simulink library "lib_TCML"  (R2015a)
settings: Solver=ode45  StartTime=0.0  StopTime=10.0  RelTol=1e-3
libraries: simulink x5
(part 6 of 7)

== matlab function lib_TCML/Dynamic Tip Clearance/Case Deformation/1D Trans Conduction model - variable props & general BCs/MATLAB Function ==
  data: k input; T output; Cp input; rho input; convin input; Tfin input; hin input; condin input; Tsin input; radin input; Textin input; uin input; convout input; Tfout input; hout input; condout input; Tsout input; radout input; Textout input; uout input; x input; a input; dt input; To input; Erro input; Err output; BN input
function [T,Err] = HeatX1D(k,Cp,rho,convin,Tfin,hin,condin,Tsin,...
    radin,Textin,uin,convout,Tfout,hout,condout,Tsout,radout,Textout,uout,...
    x,a,dt,To,Erro,BN)
%#codegen

% Written by: Jonathan Kratz, NASA GRC
% Date: August 1, 2016
%
% Description: This MATLAB function block solves a 1-D heat transfer
% problem with the potential for various boundary conditions including
% convection, conduction, and radiation. The function is capable of
% accepting time-varying thermal properties including the conductivity,
% specific heat, and density of the solid structure. Heat transfer
% coefficients can also be time-varying. The function is equiped to handle
% planor and cylindrical geometries. A generic non-uniform spatial
% discretization may be used but a constant time-step is encouraged for
% accuracy in time. The block applies a 1-D Finite Difference Method (FDM)
% to solve the equation:
%                  _                     _
%   dT     1      |  /dk   ak\ dT     d2T |
%   -- = ------ * | | -- + -- |-- + k --- |
%   dt   rho*Cp   |_ \dx    x/ dx     dx2_|
%
% This is done through the Crank-Nicolson Method in conjunction with 
% Thomas's Algorithm. The boundary conditions use linear heat transfer 
% coefficients and it is suggested that these coefficients be evaluated 
% using thermal properties of the previous time-step (i.e. temperature of 
% the structure and thermodynamic properties of the surrounding gases).
% Depending on the problem they may be assumed constant.
%
% Inputs:
% Thermal Properties:
%   k - thermal conductivity of the structure [1 x number of nodes]
%   Cp - heat capacity of the structure [1 x number of nodes]
%   rho - density of the structure [1 x number of nodes]
% Boundary Conditions:
%   Tfin - temperature of fluid on the inside surface
%   hin - convective heat transfer coefficient on the inside surface
%   Tsin - temperature of a contacting structure on the inside surface
%   Textin - temperature of a distant external radiating source/sink 
%       exposed to the inner surface
%   uin - linear radiative heat transfer coefficient between the inner
%       surface and external radiating source/sink it is exposed to
%   Tfout - temperature of fluid on the outer surface
%   hout - convective heat transfer coefficient on the outer surface
%   Tsout - temperature of a contacting structure on the outer surface
%   Textout - temperature of a distant external radiating source/sink 
%       exposed to the outer surface
%   uin - linear radiative heat transfer coefficient between the outer
%       surface and external radiating source/sink it is exposed to
% Geometry/Discretization:
%   x - discretized spatial coordinates
%   a - shape variable (0 - planar, 1 - cylindrical)
% Solver:
%   dt - time-step of the solver
%   To - initial condition for the solver/initial temperature of the
%       structure [1 x number of nodes]
% Error/Warning Detection
%   Erro - array with error states. Tracks errors/warnings that have been
%       detected.
%   BN - block name. Used in warning messages.
%  
% Discretization guidelines: The first and last nodes should be on the 
% surface. It is important that that the first node should be half the size 
% as the second node and the last node should be half the size of the 
% second to last node. This is due to the assumptions made in the 
% formulization of the boundary condition equations. Also, for planar 
% geometries the first value of the discretization array x (which 
% corresponds to the first node) can be any real numeric value (it does not
% have to be zero, equations use node size so relative position is what 
% matters). In the case of a cylindrical geometry the first value in the x 
% array should be the inner radius of the structure. It should go without 
% saying that the spatial discretization array x is required to be 
% montonically increasing.

% number of elements
n = length(x); %number of nodes

% initialize error/warning array
Err = Erro;
ErrNum = 1; %Error index

% check sizes ------------------------------------------------------------%
if length(x) < 4 && Erro(ErrNum) == 0
    Err(ErrNum) = 1;
    fprintf('warning in %s: x must be an array of length > 3\n',char(BN));
end
ErrNum = ErrNum + 1;
if length(k) ~= length(x) && Erro(ErrNum) == 0
    Err(ErrNum) = 1;
    fprintf('warning in %s: length of k must equal length of x\n',char(BN));
end
ErrNum = ErrNum + 1;
if length(Cp) ~= length(x) && Erro(ErrNum) == 0
    Err(ErrNum) = 1;
    fprintf('warning in %s: length of k must equal length of x\n',char(BN));
end
ErrNum = ErrNum + 1;
if length(rho) ~= length(x) && Erro(ErrNum) == 0
    Err(ErrNum) = 1;
    fprintf('warning in %s: length of k must equal length of x\n',char(BN));
end
ErrNum = ErrNum + 1;
if length(x) ~= length(x) && Erro(ErrNum) == 0
    Err(ErrNum) = 1;
    fprintf('warning in %s: length of k must equal length of x\n',char(BN));
end
ErrNum = ErrNum + 1;
if length(Tfin) ~= 1 && Erro(ErrNum) == 0
    Err(ErrNum) = 1;
    fprintf('warning in %s: Tfin must be a scalar\n',char(BN));
end
ErrNum = ErrNum + 1;
if length(hin) ~= 1 && Erro(ErrNum) == 0
    Err(ErrNum) = 1;
    fprintf('warning in %s: hin must be a scalar\n',char(BN));
end
ErrNum = ErrNum + 1;
if length(Tsin) ~= 1 && Erro(ErrNum) == 0
    Err(ErrNum) = 1;
    fprintf('warning in %s: Tsin must be a scalar\n',char(BN));
end
ErrNum = ErrNum + 1;
if length(Textin) ~= 1 && Erro(ErrNum) == 0
    Err(ErrNum) = 1;
    fprintf('warning in %s: Textin must be a scalar\n',char(BN));
end
ErrNum = ErrNum + 1;
if length(uin) ~= 1 && Erro(ErrNum) == 0
    Err(ErrNum) = 1;
    fprintf('warning in %s: uin must be a scalar\n',char(BN));
end
ErrNum = ErrNum + 1;
if length(Tfout) ~= 1 && Erro(ErrNum) == 0
    Err(ErrNum) = 1;
    fprintf('warning in %s: Tfout must be a scalar\n',char(BN));
end
ErrNum = ErrNum + 1;
if length(hout) ~= 1 && Erro(ErrNum) == 0
    Err(ErrNum) = 1;
    fprintf('warning in %s: hout must be a scalar\n',char(BN));
end
ErrNum = ErrNum + 1;
if length(Tsout) ~= 1 && Erro(ErrNum) == 0
    Err(ErrNum) = 1;
    fprintf('warning in %s: Tsout must be a scalar\n',char(BN));
end
ErrNum = ErrNum + 1;
if length(Textout) ~= 1 && Erro(ErrNum) == 0
    Err(ErrNum) = 1;
    fprintf('warning in %s: Textout must be a scalar\n',char(BN));
end
ErrNum = ErrNum + 1;
if length(uout) ~= 1 && Erro(ErrNum) == 0
    Err(ErrNum) = 1;
    fprintf('warning in %s: uin must be a scalar\n',char(BN));
end
ErrNum = ErrNum + 1;
if ((length(a) ~= 1) || (a ~= 0 && a ~= 1)) && Erro(ErrNum) == 0
    Err(ErrNum) = 1;
    fprintf('warning in %s: a must be a scalar equal to 0 or 1\n',char(BN));
end
ErrNum = ErrNum + 1;
if (length(dt) ~= 1 || dt <= 0) && Erro(ErrNum) == 0
    Err(ErrNum) = 1;
    fprintf('warning in %s: dt must be a positive scalar\n',char(BN));
end
ErrNum = ErrNum + 1;

% check for physical impossibilities
if min(k) <= 0 && Erro(ErrNum) == 0
    Err(ErrNum) = 1;
    fprintf('warning in %s: elements of k cannot be zero or negative\n',char(BN));
end
ErrNum = ErrNum + 1;
if min(Cp) <= 0 && Erro(ErrNum) == 0
    Err(ErrNum) = 1;
    fprintf('warning in %s: elements of Cp cannot be zero or negative\n',char(BN));
end
ErrNum = ErrNum + 1;
if min(rho) <= 0 && Erro(ErrNum) == 0
    Err(ErrNum) = 1;
    fprintf('warning in %s: elements of rho cannot be zero or negative\n',char(BN));
end
ErrNum = ErrNum + 1;
if min(To) < 0 && Erro(ErrNum) == 0
    Err(ErrNum) = 1;
    fprintf('warning in %s: elements of T0 are negative. On an absolute scale this is not possible.\n',char(BN));
end
ErrNum = ErrNum + 1;
if Tfin < 0 && Erro(ErrNum) == 0
    Err(ErrNum) = 1;
    fprintf('warning in %s: Tfin is negative. On an absolute scale this is not possible.\n',char(BN));
end
ErrNum = ErrNum + 1;
if Tfout < 0 && Erro(ErrNum) == 0
    Err(ErrNum) = 1;
    fprintf('warning in %s: Tfout is negative. On an absolute scale this is not possible.\n',char(BN));
end
ErrNum = ErrNum + 1;
if Tsin < 0 && Erro(ErrNum) == 0
    Err(ErrNum) = 1;
    fprintf('warning in %s: Tsin is negative. On an absolute scale this is not possible.\n',char(BN));
end
ErrNum = ErrNum + 1;
if Tsout < 0 && Erro(ErrNum) == 0
    Err(ErrNum) = 1;
    fprintf('warning in %s: Tsout is negative. On an absolute scale this is not possible.\n',char(BN));
end
ErrNum = ErrNum + 1;
if Textin < 0 && Erro(ErrNum) == 0
    Err(ErrNum) = 1;
    fprintf('warning in %s: Textin is negative. On an absolute scale this is not possible.\n',char(BN));
end
ErrNum = ErrNum + 1;
if Textout < 0 && Erro(ErrNum) == 0
    Err(ErrNum) = 1;
    fprintf('warning in %s: Textout is negative. On an absolute scale this is not possible.\n',char(BN));
end
ErrNum = ErrNum + 1;
if hin < 0 && Erro(ErrNum) == 0
    Err(ErrNum) = 1;
    fprintf('warning in %s: hin must be positive.\n',char(BN));
end
ErrNum = ErrNum + 1;
if hout < 0 && Erro(ErrNum) == 0
    Err(ErrNum) = 1;
    fprintf('warning in %s: hout must be positive.\n',char(BN));
end
ErrNum = ErrNum + 1;
if uin < 0 && Erro(ErrNum) == 0
    Err(ErrNum) = 1;
    fprintf('warning in %s: uin must be positive.\n',char(BN));
end
ErrNum = ErrNum + 1;
if uout < 0 && Erro(ErrNum) == 0
    Err(ErrNum) = 1;
    fprintf('warning in %s: uout must be positive.\n',char(BN));
end
ErrNum = ErrNum + 1;

% check for defiance of block constraints
diffx = diff(x);
if min(diffx) <= 0 && Erro(ErrNum) == 0
    Err(ErrNum) = 1;
    fprintf('warning in %s: x must be monotonically increasing\n',char(BN));
end
ErrNum = ErrNum + 1;
if (x(2)-x(1))-(x(3)-x(2)) >= 10^-5 && Erro(ErrNum) == 0
    Err(ErrNum) = 1;
    fprintf('warning in %s: the first node may not be half the thickness of the\nneighboring interior node as is required for planar geometries in the\nequation formulation of this block. To assure the first node is\nof the appropriate size assure (x(2)-x(1))-(x(3)-x(2)) = 0.\n',char(BN));
end
ErrNum = ErrNum + 1;
if (x(n)-x(n-1))-(x(n-1)-x(n-2)) >= 10^-5 && Erro(ErrNum) == 0
    Err(ErrNum) = 1;
    fprintf('warning in %s: the last node may not be half the thickness of the\nneighboring interior node as is required for planar geometries in the\nequation formulation of this block. To assure the last node is\nof the appropriate size assure (x(n)-x(n-1))-(x(n-1)-x(n-2)) = 0\nwhere n is the total number of nodes.\n',char(BN));
end
ErrNum = ErrNum + 1;
if a == 1 && x(1) < 10^-6 %protect against dividing by zero
    if Erro(ErrNum) == 0
        fprintf('warning in %s: x(1) is close to zero, value changed to 10^-6 to prevent dividing by zero\n',char(BN));
    end
    Err(ErrNum) = 1;
    x(1) = 10^-6;
end
ErrNum = ErrNum + 1;

% verify at least one BC type is active for each surface
if condin == 0 && convin == 0 && radin == 0 && Erro(ErrNum) == 0
    fprintf('warning in %s: at least one boundary condition type (convection, radiation, conduction) must be active for the inner surface\n',char(BN));
    Err(ErrNum) = 1;
end
ErrNum = ErrNum + 1;
% verify at least one BC type is active for each surface
if condout == 0 && convout == 0 && radout == 0 && Erro(ErrNum) == 0
    fprintf('warning in %s: at least one boundary condition type (convection, radiation, conduction) must be active for the outer surface\n',char(BN));
    Err(ErrNum) = 1;
end

% make external convection at boundaries zero if there is no convection BC
if convin == 0
    hin = 0;
end
if convout == 0
    hout = 0;
end

% make external radiation at boundaries zero if there is no radiation BC
if radin == 0
    uin = 0;
end
if radout == 0
    uout = 0;
end

% form system of equations in tridiagonal arrays -------------------------%
%  _                                 _  _   _     _   _ 
% | D1   A1   0    .    .    .    0   || T1  |   | C1  |
% | B1   D2   A2   0              .   || T2  |   | C2  |
% | 0    B2   D3   A3   .         .   || T3  |   | C3  |
% | .    0    .    .    .    .    .   || .   | = | .   |
% | .         .    .    .    .    0   || .   |   | .   | 
% | .              .    Bn-2 Dn-1 An-1|| Tn-1|   | Cn-1|
% |_0    .    .    .    0    Bn-1 Dn _||_Tn _|   |_Cn _|
%
% Initialize system arrays B, D, A, and C
B = zeros(1,n); %initialize B array
D = zeros(1,n); %initialize D array
A = zeros(1,n); %initialize A array
C = zeros(1,n); %initialize C array
% node thickness
dx = zeros(1,n); %initialize dx array
for i = 1:n
    if i == 1
        dx(i) = (x(2)-x(1));
    elseif i == n
        dx(i) = (x(n)-x(n-1));
    else
        del1 = x(i) - x(i-1);
        dx(i) = 2*del1 - dx(i-1);
    end
end
% --- inner node (half size of interior node with point on surface)
Fo1 = 0; %Fourier number
Bi1 = 0; %Boit number
BiRad1 = 0; %analogous Boit number for radiation
Fos1 = 0; %Fourier number for conduction BC
dx1 = x(2) - x(1); %node size
% planar
if a == 0
    Fo1 = dt*k(1)/(rho(1)*Cp(1)*dx1^2); %Fourier number
    Bi1 = hin*dx1/k(1); %Boit number
    BiRad1 = uin*dx1/k(1); %analogous Boit number for radiation
    if condin == 0
        Fos1 = 0;
    else
        Fos1 = Fo1; %Fourier number for conduction BC
    end
end
% cylindrical
if a == 1
    Fo1 = dt*k(1)/(rho(1)*Cp(1)*((x(2)-dx1/2)^2-x(1)^2)*log(x(2)/x(1))); %Fourier number
    Bi1 = hin*x(1)*log(x(2)/x(1))/k(1); %Boit number
    BiRad1 = uin*x(1)*log(x(2)/x(1))/k(1); %analogous Boit number for radiation
    if condin == 0
        Fos1 = 0;
    else
        if (x(1)-dx1) <= 0
            dx1 = 0;
        end
        Fos1 = dt*k(1)/(rho(1)*Cp(1)*((x(2)-dx1/2)^2-x(1)^2)*log((x(1)/(x(1)-dx1)))); %Fourier number for conduction BC
    end
end
% form system arrays
B(1) = 0;
D(1) = 1 + Fo1 + Fo1*Bi1 + Fo1*BiRad1 + Fos1; %system array D
A(1) = -Fo1; %system array A
C(1) = (1 - Fo1 - Fo1*Bi1 - Fo1*BiRad1 - Fos1)*To(1) + Fo1*To(2) + 2*Fo1*Bi1*Tfin + 2*Fo1*BiRad1*Textin + 2*Fos1*Tsin; %system array C
% --- interior nodes
for i = 2:(n-1)
    % distance between nodes
    del1 = x(i) - x(i-1);
    del2 = x(i+1) - x(i);
    % simplification coefficients (for spatial discretization)
    C1 = 1 + (del1^3/del2^2 - del1)/(del2 + del1);
    C2 = 1 + (del1/del2)^3;
    C3 = (del1/del2)^3 - ((del1^3/del2^2) - del1)/(del2+del1);
    % calculated Fourier numbers
    Fo = 2*k(i)*dt/(rho(i)*Cp(i)*(del1^2 + del1^3/del2)); %Fourier number
    Fok = (dt/(rho(i)*Cp(i)*(del1+del2)))*((k(i+1)-k(i-1))/(del1+del2) + a*k(i)/x(i)); %Fourier number for conductivity variation and shape
    % adjust equations for change in materials
    %   when there is a change in materials the transition in materials
    %   properties, most notabely thermal conductivity, is abrupt. This
    %   discontinuty can cause accuracy and stability issues with the 
    %   derivative term dk/dt = (k(i+1)-k(i-1))/(del1+del2). Therefore a
    %   more robust approach is utilized when a material transition is
    %   detected. This method is document in "Integrated Turbine Tip
    %   Clearance and Gas Turbine Engine Simulation" by J. Chapman, J.
    %   Kratz, T.-H. Guo, and J. Litt. The method uses a transition Fourier
    %   number to address the discontinuity. The method from this reference
    %   has been generalized for non-uniform discretizations and geometries
    %   that could be either planar or cylindrical. When there is not a
    %   transition in materials the dk/dt term should be better
    %   approximated with the central difference scheme that is used and
    %   the standard formulation will be utilized. Material transition is
    %   detected by a sigificant (10%) increase or decrease in thermal 
    %   conductivity.
    if (k(i+1)/k(i)) > 1.1 || (k(i+1)/k(i)) < 0.9 %detect change in material
        Fo = k(i)*dt/(rho(i)*Cp(i)*dx(i)^2);
        Fok = (dt/(rho(i)*Cp(i)*(del1+del2)))*(a*k(i)/x(i));
        Fob = (k(i)*(dx(i)/2)+k(i+1)*(del2-dx(i)/2))*dt/(rho(i)*Cp(i)*del2*del1*del2);
        K1 = Fo;
        K2 = 2*0.5*(Fo+Fob); 
        K3 = Fob;
    elseif (k(i)/k(i-1)) > 1.1 || (k(i)/k(i-1)) < 0.9 %detect change in material
        Fo = k(i)*dt/(rho(i)*Cp(i)*dx(i)^2);
        Fok = (dt/(rho(i)*Cp(i)*(del1+del2)))*(a*k(i)/x(i));
        Foa = (k(i)*(dx(i)/2)+k(i-1)*(del1-dx(i)/2))*dt/(rho(i)*Cp(i)*del1*del1*del2);
        K1 = Foa;
        K2 = 2*0.5*(Fo+Foa); 
        K3 = Fo;
    else % no change in material detected - go with standard solution
        K1 = C1*Fo;
        K2 = C2*Fo;
        K3 = C3*Fo;
    end
    % form system arrays (B, D, A, and C)
    B(i) = 0.5*Fok - 0.5*K1;
    D(i) = 1 + 0.5*K2;
    A(i) = -0.5*Fok - 0.5*K3;
    C(i) = (-0.5*Fok+0.5*K1)*To(i-1) + (1-0.5*K2)*To(i) + (0.5*Fok+0.5*K3)*To(i+1);
end
% --- outer node (half size of interior node with point on surface)
Fon = 0; %Fourier number
Bin = 0; %Boit number
BiRadn = 0; %analogous Boit number for radiation
Fosn = 0; %Fourier number for conduction BC
dxn = x(n) - x(n-1); %node size
% planar
if a == 0
    Fon = dt*k(n)/(rho(n)*Cp(n)*dxn^2); %Fourier number
    Bin = hout*dxn/k(n); %Boit number
    BiRadn = uout*dxn/k(n); %analogous Boit number for radiation
    if condout == 0
        Fosn = 0;
    else
        Fosn = Fon; %Fourier number for conduction BC
    end
end
% cylindrical
if a == 1
    Fon = dt*k(n)/(rho(n)*Cp(n)*(x(n)^2-(x(n-1)+dxn/2)^2)*log(x(n)/x(n-1))); %Fourier number
    Bin = hout*x(n)*log(x(n)/x(n-1))/k(n); %Boit number
    BiRadn = uout*x(n)*log(x(n)/x(n-1))/k(n); %analogous Boit number for radiation
    if condout == 0
        Fosn = 0;
    else
        Fosn = dt*k(n)/(rho(n)*Cp(n)*(x(n)^2-(x(n-1)+dxn/2)^2)*log((x(n)+dxn)/x(n))); %Fourier number for conduction BC
    end
end
% form system arrays
D(n) = 1 + Fon + Fon*Bin + Fon*BiRadn + Fosn; %system array D
B(n) = -Fon; %system array B
A(n) = 0; %system array A
C(n) = (1 - Fon - Fon*Bin - Fon*BiRadn - Fosn)*To(n) + Fon*To(n-1) + 2*Fon*Bin*Tfout + 2*Fon*BiRadn*Textout + 2*Fosn*Tsout; %system array C

% solve for new temperatures using Thomas's Algorithm --------------------%
Dnew = zeros(1,n);
Cnew = zeros(1,n);
Dnew(1) = D(1);
Cnew(1) = C(1);
% build the rest of the new D-vector and C-vector using Guassian
% elimination
for i = 2:n
    Dnew(i) = D(i) - A(i-1)*B(i)/Dnew(i-1);
    Cnew(i) = C(i) - B(i)*Cnew(i-1)/Dnew(i-1);
end
% initialize the solution vector (i.e. the new temperature vector T)
T = zeros(1,n);
T(n) = Cnew(n)/Dnew(n);
for i = (n-1):-1:1
    T(i) = (Cnew(i) - A(i)*T(i+1))/Dnew(i);
end

== matlab function lib_TCML/Dynamic Tip Clearance/Case Deformation/Deformation1/Thermal Expansion 1D Elastic/MATLAB Function ==
  data: T_data input; L output; alpha_data input; Lo input; To input; Tf input; Erro input; BN input; Err output
function [L,Err] = ThermalExpansion(T_data,alpha_data,Lo,To,Tf,Erro,BN)
%#codegen

% initialize error/warning array
Err = Erro;
ErrNum = 1; %Error index

% number of data points for interpolation and numerical integration
n = 50;

%check input sizes
if length(T_data) < 2 && Erro(ErrNum) == 0
    Err(ErrNum) = 1;
    fprintf('warning in %s: The temperature data array (T_data) must be an array of at least 2 elements\n',char(BN));
end
ErrNum = ErrNum + 1;
if length(T_data) ~= length(alpha_data) && Erro(ErrNum) == 0
    Err(ErrNum) = 1;
    fprintf('warning in %s: The temperature data array (T_data) and corresponding thermal expansion coefficient data array (alpha_data) must be the same size\n',char(BN));
end
ErrNum = ErrNum + 1;
    
%check that To and Tf are in the range of T_data
if To < min(T_data)
    To = min(T_data);
    Err(ErrNum) = 1;
    if Erro(ErrNum) == 0
        fprintf('warning in %s: The previous/reference temperature (To) is less than the minimum value of the temperature data array T_data. Expand the data arrays to assure good results. The previous/reference temperature (To) has been set to the minimum value of T_data to avoid errors.\n',char(BN));
    end
end
ErrNum = ErrNum + 1;
if To > max(T_data)
    To = max(T_data);
    Err(ErrNum) = 1;
    if Erro(ErrNum) == 0
        fprintf('warning in %s: The previous/reference temperature (To) is greater than the maximum value of the temperature data array T_data. Expand the data arrays to assure good results. The previous/reference temperature (To) has been set to the maximum value of T_data to avoid errors.\n',char(BN));
    end
end
ErrNum = ErrNum + 1;
if Tf < min(T_data)
    Tf = min(T_data);
    Err(ErrNum) = 1;
    if Erro(ErrNum) == 0
        fprintf('warning in %s: The current temperature (Tf) is less than the minimum value of the temperature data array T_data. Expand the data arrays to assure good results. The current temperature (Tf) has been set to the maximum value of T_data to avoid errors.\n',char(BN));
    end
end
ErrNum = ErrNum + 1;
if Tf > max(T_data)
    Tf = max(T_data);
    Err(ErrNum) = 1;
    if Erro(ErrNum) == 0
        fprintf('warning in %s: The current temperature (Tf) is greater than the maximum value of the temperature data array T_data. Expand the data arrays to assure good results. The current temperature (Tf) has been set to the maximum value of T_data to avoid errors.\n',char(BN));
    end
end
ErrNum = ErrNum + 1;

%check that T_data is monotonically increasing
diffT = diff(T_data);
if min(diffT) <= 0 && Erro(ErrNum) == 0
    Err(ErrNum) = 1;
    fprintf('warning in %s: The temperature data array (T_data) must be monotonically increasing\n',char(BN));
end

T = linspace(To,Tf,n);
alpha = zeros(1,n);
for i = 1:n
    alpha(i) = interp1(T_data,alpha_data,T(i),'linear');
end

Int_alphadT = trapz(T,alpha);
dL = Lo*Int_alphadT;

L = Lo + dL;

== matlab function lib_TCML/Dynamic Tip Clearance/Blade Deformation/Deformation/Deformation Due To Thermal Expansion/Thermal Expansion 1D Elastic/MATLAB Function ==
  data: T_data input; L output; alpha_data input; Lo input; To input; Tf input; Erro input; BN input; Err output
function [L,Err] = ThermalExpansion(T_data,alpha_data,Lo,To,Tf,Erro,BN)
%#codegen

% initialize error/warning array
Err = Erro;
ErrNum = 1; %Error index

% number of data points for interpolation and numerical integration
n = 50;

%check input sizes
if length(T_data) < 2 && Erro(ErrNum) == 0
    Err(ErrNum) = 1;
    fprintf('warning in %s: The temperature data array (T_data) must be an array of at least 2 elements\n',char(BN));
end
ErrNum = ErrNum + 1;
if length(T_data) ~= length(alpha_data) && Erro(ErrNum) == 0
    Err(ErrNum) = 1;
    fprintf('warning in %s: The temperature data array (T_data) and corresponding thermal expansion coefficient data array (alpha_data) must be the same size\n',char(BN));
end
ErrNum = ErrNum + 1;
    
%check that To and Tf are in the range of T_data
if To < min(T_data)
    To = min(T_data);
    Err(ErrNum) = 1;
    if Erro(ErrNum) == 0
        fprintf('warning in %s: The previous/reference temperature (To) is less than the minimum value of the temperature data array T_data. Expand the data arrays to assure good results. The previous/reference temperature (To) has been set to the minimum value of T_data to avoid errors.\n',char(BN));
    end
end
ErrNum = ErrNum + 1;
if To > max(T_data)
    To = max(T_data);
    Err(ErrNum) = 1;
    if Erro(ErrNum) == 0
        fprintf('warning in %s: The previous/reference temperature (To) is greater than the maximum value of the temperature data array T_data. Expand the data arrays to assure good results. The previous/reference temperature (To) has been set to the maximum value of T_data to avoid errors.\n',char(BN));
    end
end
ErrNum = ErrNum + 1;
if Tf < min(T_data)
    Tf = min(T_data);
    Err(ErrNum) = 1;
    if Erro(ErrNum) == 0
        fprintf('warning in %s: The current temperature (Tf) is less than the minimum value of the temperature data array T_data. Expand the data arrays to assure good results. The current temperature (Tf) has been set to the maximum value of T_data to avoid errors.\n',char(BN));
    end
end
ErrNum = ErrNum + 1;
if Tf > max(T_data)
    Tf = max(T_data);
    Err(ErrNum) = 1;
    if Erro(ErrNum) == 0
        fprintf('warning in %s: The current temperature (Tf) is greater than the maximum value of the temperature data array T_data. Expand the data arrays to assure good results. The current temperature (Tf) has been set to the maximum value of T_data to avoid errors.\n',char(BN));
    end
end
ErrNum = ErrNum + 1;

%check that T_data is monotonically increasing
diffT = diff(T_data);
if min(diffT) <= 0 && Erro(ErrNum) == 0
    Err(ErrNum) = 1;
    fprintf('warning in %s: The temperature data array (T_data) must be monotonically increasing\n',char(BN));
end

T = linspace(To,Tf,n);
alpha = zeros(1,n);
for i = 1:n
    alpha(i) = interp1(T_data,alpha_data,T(i),'linear');
end

Int_alphadT = trapz(T,alpha);
dL = Lo*Int_alphadT;

L = Lo + dL;

== matlab function lib_TCML/Dynamic Tip Clearance/Blade Deformation/Deformation1/Deformation Due To Thermal Expansion/Thermal Expansion 1D Elastic/MATLAB Function ==
  data: T_data input; L output; alpha_data input; Lo input; To input; Tf input; Erro input; BN input; Err output
function [L,Err] = ThermalExpansion(T_data,alpha_data,Lo,To,Tf,Erro,BN)
%#codegen

% initialize error/warning array
Err = Erro;
ErrNum = 1; %Error index

% number of data points for interpolation and numerical integration
n = 50;

%check input sizes
if length(T_data) < 2 && Erro(ErrNum) == 0
    Err(ErrNum) = 1;
    fprintf('warning in %s: The temperature data array (T_data) must be an array of at least 2 elements\n',char(BN));
end
ErrNum = ErrNum + 1;
if length(T_data) ~= length(alpha_data) && Erro(ErrNum) == 0
    Err(ErrNum) = 1;
    fprintf('warning in %s: The temperature data array (T_data) and corresponding thermal expansion coefficient data array (alpha_data) must be the same size\n',char(BN));
end
ErrNum = ErrNum + 1;
    
%check that To and Tf are in the range of T_data
if To < min(T_data)
    To = min(T_data);
    Err(ErrNum) = 1;
    if Erro(ErrNum) == 0
        fprintf('warning in %s: The previous/reference temperature (To) is less than the minimum value of the temperature data array T_data. Expand the data arrays to assure good results. The previous/reference temperature (To) has been set to the minimum value of T_data to avoid errors.\n',char(BN));
    end
end
ErrNum = ErrNum + 1;
if To > max(T_data)
    To = max(T_data);
    Err(ErrNum) = 1;
    if Erro(ErrNum) == 0
        fprintf('warning in %s: The previous/reference temperature (To) is greater than the maximum value of the temperature data array T_data. Expand the data arrays to assure good results. The previous/reference temperature (To) has been set to the maximum value of T_data to avoid errors.\n',char(BN));
    end
end
ErrNum = ErrNum + 1;
if Tf < min(T_data)
    Tf = min(T_data);
    Err(ErrNum) = 1;
    if Erro(ErrNum) == 0
        fprintf('warning in %s: The current temperature (Tf) is less than the minimum value of the temperature data array T_data. Expand the data arrays to assure good results. The current temperature (Tf) has been set to the maximum value of T_data to avoid errors.\n',char(BN));
    end
end
ErrNum = ErrNum + 1;
if Tf > max(T_data)
    Tf = max(T_data);
    Err(ErrNum) = 1;
    if Erro(ErrNum) == 0
        fprintf('warning in %s: The current temperature (Tf) is greater than the maximum value of the temperature data array T_data. Expand the data arrays to assure good results. The current temperature (Tf) has been set to the maximum value of T_data to avoid errors.\n',char(BN));
    end
end
ErrNum = ErrNum + 1;

%check that T_data is monotonically increasing
diffT = diff(T_data);
if min(diffT) <= 0 && Erro(ErrNum) == 0
    Err(ErrNum) = 1;
    fprintf('warning in %s: The temperature data array (T_data) must be monotonically increasing\n',char(BN));
end

T = linspace(To,Tf,n);
alpha = zeros(1,n);
for i = 1:n
    alpha(i) = interp1(T_data,alpha_data,T(i),'linear');
end

Int_alphadT = trapz(T,alpha);
dL = Lo*Int_alphadT;

L = Lo + dL;

== matlab function lib_TCML/Dynamic Tip Clearance/Rotor Deformation/1D Trans Conduction model - variable props & general BCs/MATLAB Function ==
  data: k input; T output; Cp input; rho input; convin input; Tfin input; hin input; condin input; Tsin input; radin input; Textin input; uin input; convout input; Tfout input; hout input; condout input; Tsout input; radout input; Textout input; uout input; x input; a input; dt input; To input; Erro input; Err output; BN input
function [T,Err] = HeatX1D(k,Cp,rho,convin,Tfin,hin,condin,Tsin,...
    radin,Textin,uin,convout,Tfout,hout,condout,Tsout,radout,Textout,uout,...
    x,a,dt,To,Erro,BN)
%#codegen

% Written by: Jonathan Kratz, NASA GRC
% Date: August 1, 2016
%
% Description: This MATLAB function block solves a 1-D heat transfer
% problem with the potential for various boundary conditions including
% convection, conduction, and radiation. The function is capable of
% accepting time-varying thermal properties including the conductivity,
% specific heat, and density of the solid structure. Heat transfer
% coefficients can also be time-varying. The function is equiped to handle
% planor and cylindrical geometries. A generic non-uniform spatial
% discretization may be used but a constant time-step is encouraged for
% accuracy in time. The block applies a 1-D Finite Difference Method (FDM)
% to solve the equation:
%                  _                     _
%   dT     1      |  /dk   ak\ dT     d2T |
%   -- = ------ * | | -- + -- |-- + k --- |
%   dt   rho*Cp   |_ \dx    x/ dx     dx2_|
%
% This is done through the Crank-Nicolson Method in conjunction with 
% Thomas's Algorithm. The boundary conditions use linear heat transfer 
% coefficients and it is suggested that these coefficients be evaluated 
% using thermal properties of the previous time-step (i.e. temperature of 
% the structure and thermodynamic properties of the surrounding gases).
% Depending on the problem they may be assumed constant.
%
% Inputs:
% Thermal Properties:
%   k - thermal conductivity of the structure [1 x number of nodes]
%   Cp - heat capacity of the structure [1 x number of nodes]
%   rho - density of the structure [1 x number of nodes]
% Boundary Conditions:
%   Tfin - temperature of fluid on the inside surface
%   hin - convective heat transfer coefficient on the inside surface
%   Tsin - temperature of a contacting structure on the inside surface
%   Textin - temperature of a distant external radiating source/sink 
%       exposed to the inner surface
%   uin - linear radiative heat transfer coefficient between the inner
%       surface and external radiating source/sink it is exposed to
%   Tfout - temperature of fluid on the outer surface
%   hout - convective heat transfer coefficient on the outer surface
%   Tsout - temperature of a contacting structure on the outer surface
%   Textout - temperature of a distant external radiating source/sink 
%       exposed to the outer surface
%   uin - linear radiative heat transfer coefficient between the outer
%       surface and external radiating source/sink it is exposed to
% Geometry/Discretization:
%   x - discretized spatial coordinates
%   a - shape variable (0 - planar, 1 - cylindrical)
% Solver:
%   dt - time-step of the solver
%   To - initial condition for the solver/initial temperature of the
%       structure [1 x number of nodes]
% Error/Warning Detection
%   Erro - array with error states. Tracks errors/warnings that have been
%       detected.
%   BN - block name. Used in warning messages.
%  
% Discretization guidelines: The first and last nodes should be on the 
% surface. It is important that that the first node should be half the size 
% as the second node and the last node should be half the size of the 
% second to last node. This is due to the assumptions made in the 
% formulization of the boundary condition equations. Also, for planar 
% geometries the first value of the discretization array x (which 
% corresponds to the first node) can be any real numeric value (it does not
% have to be zero, equations use node size so relative position is what 
% matters). In the case of a cylindrical geometry the first value in the x 
% array should be the inner radius of the structure. It should go without 
% saying that the spatial discretization array x is required to be 
% montonically increasing.

% number of elements
n = length(x); %number of nodes

% initialize error/warning array
Err = Erro;
ErrNum = 1; %Error index

% check sizes ------------------------------------------------------------%
if length(x) < 4 && Erro(ErrNum) == 0
    Err(ErrNum) = 1;
    fprintf('warning in %s: x must be an array of length > 3\n',char(BN));
end
ErrNum = ErrNum + 1;
if length(k) ~= length(x) && Erro(ErrNum) == 0
    Err(ErrNum) = 1;
    fprintf('warning in %s: length of k must equal length of x\n',char(BN));
end
ErrNum = ErrNum + 1;
if length(Cp) ~= length(x) && Erro(ErrNum) == 0
    Err(ErrNum) = 1;
    fprintf('warning in %s: length of k must equal length of x\n',char(BN));
end
ErrNum = ErrNum + 1;
if length(rho) ~= length(x) && Erro(ErrNum) == 0
    Err(ErrNum) = 1;
    fprintf('warning in %s: length of k must equal length of x\n',char(BN));
end
ErrNum = ErrNum + 1;
if length(x) ~= length(x) && Erro(ErrNum) == 0
    Err(ErrNum) = 1;
    fprintf('warning in %s: length of k must equal length of x\n',char(BN));
end
ErrNum = ErrNum + 1;
if length(Tfin) ~= 1 && Erro(ErrNum) == 0
    Err(ErrNum) = 1;
    fprintf('warning in %s: Tfin must be a scalar\n',char(BN));
end
ErrNum = ErrNum + 1;
if length(hin) ~= 1 && Erro(ErrNum) == 0
    Err(ErrNum) = 1;
    fprintf('warning in %s: hin must be a scalar\n',char(BN));
end
ErrNum = ErrNum + 1;
if length(Tsin) ~= 1 && Erro(ErrNum) == 0
    Err(ErrNum) = 1;
    fprintf('warning in %s: Tsin must be a scalar\n',char(BN));
end
ErrNum = ErrNum + 1;
if length(Textin) ~= 1 && Erro(ErrNum) == 0
    Err(ErrNum) = 1;
    fprintf('warning in %s: Textin must be a scalar\n',char(BN));
end
ErrNum = ErrNum + 1;
if length(uin) ~= 1 && Erro(ErrNum) == 0
    Err(ErrNum) = 1;
    fprintf('warning in %s: uin must be a scalar\n',char(BN));
end
ErrNum = ErrNum + 1;
if length(Tfout) ~= 1 && Erro(ErrNum) == 0
    Err(ErrNum) = 1;
    fprintf('warning in %s: Tfout must be a scalar\n',char(BN));
end
ErrNum = ErrNum + 1;
if length(hout) ~= 1 && Erro(ErrNum) == 0
    Err(ErrNum) = 1;
    fprintf('warning in %s: hout must be a scalar\n',char(BN));
end
ErrNum = ErrNum + 1;
if length(Tsout) ~= 1 && Erro(ErrNum) == 0
    Err(ErrNum) = 1;
    fprintf('warning in %s: Tsout must be a scalar\n',char(BN));
end
ErrNum = ErrNum + 1;
if length(Textout) ~= 1 && Erro(ErrNum) == 0
    Err(ErrNum) = 1;
    fprintf('warning in %s: Textout must be a scalar\n',char(BN));
end
ErrNum = ErrNum + 1;
if length(uout) ~= 1 && Erro(ErrNum) == 0
    Err(ErrNum) = 1;
    fprintf('warning in %s: uin must be a scalar\n',char(BN));
end
ErrNum = ErrNum + 1;
if ((length(a) ~= 1) || (a ~= 0 && a ~= 1)) && Erro(ErrNum) == 0
    Err(ErrNum) = 1;
    fprintf('warning in %s: a must be a scalar equal to 0 or 1\n',char(BN));
end
ErrNum = ErrNum + 1;
if (length(dt) ~= 1 || dt <= 0) && Erro(ErrNum) == 0
    Err(ErrNum) = 1;
    fprintf('warning in %s: dt must be a positive scalar\n',char(BN));
end
ErrNum = ErrNum + 1;

% check for physical impossibilities
if min(k) <= 0 && Erro(ErrNum) == 0
    Err(ErrNum) = 1;
    fprintf('warning in %s: elements of k cannot be zero or negative\n',char(BN));
end
ErrNum = ErrNum + 1;
if min(Cp) <= 0 && Erro(ErrNum) == 0
    Err(ErrNum) = 1;
    fprintf('warning in %s: elements of Cp cannot be zero or negative\n',char(BN));
end
ErrNum = ErrNum + 1;
if min(rho) <= 0 && Erro(ErrNum) == 0
    Err(ErrNum) = 1;
    fprintf('warning in %s: elements of rho cannot be zero or negative\n',char(BN));
end
ErrNum = ErrNum + 1;
if min(To) < 0 && Erro(ErrNum) == 0
    Err(ErrNum) = 1;
    fprintf('warning in %s: elements of T0 are negative. On an absolute scale this is not possible.\n',char(BN));
end
ErrNum = ErrNum + 1;
if Tfin < 0 && Erro(ErrNum) == 0
    Err(ErrNum) = 1;
    fprintf('warning in %s: Tfin is negative. On an absolute scale this is not possible.\n',char(BN));
end
ErrNum = ErrNum + 1;
if Tfout < 0 && Erro(ErrNum) == 0
    Err(ErrNum) = 1;
    fprintf('warning in %s: Tfout is negative. On an absolute scale this is not possible.\n',char(BN));
end
ErrNum = ErrNum + 1;
if Tsin < 0 && Erro(ErrNum) == 0
    Err(ErrNum) = 1;
    fprintf('warning in %s: Tsin is negative. On an absolute scale this is not possible.\n',char(BN));
end
ErrNum = ErrNum + 1;
if Tsout < 0 && Erro(ErrNum) == 0
    Err(ErrNum) = 1;
    fprintf('warning in %s: Tsout is negative. On an absolute scale this is not possible.\n',char(BN));
end
ErrNum = ErrNum + 1;
if Textin < 0 && Erro(ErrNum) == 0
    Err(ErrNum) = 1;
    fprintf('warning in %s: Textin is negative. On an absolute scale this is not possible.\n',char(BN));
end
ErrNum = ErrNum + 1;
if Textout < 0 && Erro(ErrNum) == 0
    Err(ErrNum) = 1;
    fprintf('warning in %s: Textout is negative. On an absolute scale this is not possible.\n',char(BN));
end
ErrNum = ErrNum + 1;
if hin < 0 && Erro(ErrNum) == 0
    Err(ErrNum) = 1;
    fprintf('warning in %s: hin must be positive.\n',char(BN));
end
ErrNum = ErrNum + 1;
if hout < 0 && Erro(ErrNum) == 0
    Err(ErrNum) = 1;
    fprintf('warning in %s: hout must be positive.\n',char(BN));
end
ErrNum = ErrNum + 1;
if uin < 0 && Erro(ErrNum) == 0
    Err(ErrNum) = 1;
    fprintf('warning in %s: uin must be positive.\n',char(BN));
end
ErrNum = ErrNum + 1;
if uout < 0 && Erro(ErrNum) == 0
    Err(ErrNum) = 1;
    fprintf('warning in %s: uout must be positive.\n',char(BN));
end
ErrNum = ErrNum + 1;

% check for defiance of block constraints
diffx = diff(x);
if min(diffx) <= 0 && Erro(ErrNum) == 0
    Err(ErrNum) = 1;
    fprintf('warning in %s: x must be monotonically increasing\n',char(BN));
end
ErrNum = ErrNum + 1;
if (x(2)-x(1))-(x(3)-x(2)) >= 10^-5 && Erro(ErrNum) == 0
    Err(ErrNum) = 1;
    fprintf('warning in %s: the first node may not be half the thickness of the\nneighboring interior node as is required for planar geometries in the\nequation formulation of this block. To assure the first node is\nof the appropriate size assure (x(2)-x(1))-(x(3)-x(2)) = 0.\n',char(BN));
end
ErrNum = ErrNum + 1;
if (x(n)-x(n-1))-(x(n-1)-x(n-2)) >= 10^-5 && Erro(ErrNum) == 0
    Err(ErrNum) = 1;
    fprintf('warning in %s: the last node may not be half the thickness of the\nneighboring interior node as is required for planar geometries in the\nequation formulation of this block. To assure the last node is\nof the appropriate size assure (x(n)-x(n-1))-(x(n-1)-x(n-2)) = 0\nwhere n is the total number of nodes.\n',char(BN));
end
ErrNum = ErrNum + 1;
if a == 1 && x(1) < 10^-6 %protect against dividing by zero
    if Erro(ErrNum) == 0
        fprintf('warning in %s: x(1) is close to zero, value changed to 10^-6 to prevent dividing by zero\n',char(BN));
    end
    Err(ErrNum) = 1;
    x(1) = 10^-6;
end
ErrNum = ErrNum + 1;

% verify at least one BC type is active for each surface
if condin == 0 && convin == 0 && radin == 0 && Erro(ErrNum) == 0
    fprintf('warning in %s: at least one boundary condition type (convection, radiation, conduction) must be active for the inner surface\n',char(BN));
    Err(ErrNum) = 1;
end
ErrNum = ErrNum + 1;
% verify at least one BC type is active for each surface
if condout == 0 && convout == 0 && radout == 0 && Erro(ErrNum) == 0
    fprintf('warning in %s: at least one boundary condition type (convection, radiation, conduction) must be active for the outer surface\n',char(BN));
    Err(ErrNum) = 1;
end

% make external convection at boundaries zero if there is no convection BC
if convin == 0
    hin = 0;
end
if convout == 0
    hout = 0;
end

% make external radiation at boundaries zero if there is no radiation BC
if radin == 0
    uin = 0;
end
if radout == 0
    uout = 0;
end

% form system of equations in tridiagonal arrays -------------------------%
%  _                                 _  _   _     _   _ 
% | D1   A1   0    .    .    .    0   || T1  |   | C1  |
% | B1   D2   A2   0              .   || T2  |   | C2  |
% | 0    B2   D3   A3   .         .   || T3  |   | C3  |
% | .    0    .    .    .    .    .   || .   | = | .   |
% | .         .    .    .    .    0   || .   |   | .   | 
% | .              .    Bn-2 Dn-1 An-1|| Tn-1|   | Cn-1|
% |_0    .    .    .    0    Bn-1 Dn _||_Tn _|   |_Cn _|
%
% Initialize system arrays B, D, A, and C
B = zeros(1,n); %initialize B array
D = zeros(1,n); %initialize D array
A = zeros(1,n); %initialize A array
C = zeros(1,n); %initialize C array
% node thickness
dx = zeros(1,n); %initialize dx array
for i = 1:n
    if i == 1
        dx(i) = (x(2)-x(1));
    elseif i == n
        dx(i) = (x(n)-x(n-1));
    else
        del1 = x(i) - x(i-1);
        dx(i) = 2*del1 - dx(i-1);
    end
end
% --- inner node (half size of interior node with point on surface)
Fo1 = 0; %Fourier number
Bi1 = 0; %Boit number
BiRad1 = 0; %analogous Boit number for radiation
Fos1 = 0; %Fourier number for conduction BC
dx1 = x(2) - x(1); %node size
% planar
if a == 0
    Fo1 = dt*k(1)/(rho(1)*Cp(1)*dx1^2); %Fourier number
    Bi1 = hin*dx1/k(1); %Boit number
    BiRad1 = uin*dx1/k(1); %analogous Boit number for radiation
    if condin == 0
        Fos1 = 0;
    else
        Fos1 = Fo1; %Fourier number for conduction BC
    end
end
% cylindrical
if a == 1
    Fo1 = dt*k(1)/(rho(1)*Cp(1)*((x(2)-dx1/2)^2-x(1)^2)*log(x(2)/x(1))); %Fourier number
    Bi1 = hin*x(1)*log(x(2)/x(1))/k(1); %Boit number
    BiRad1 = uin*x(1)*log(x(2)/x(1))/k(1); %analogous Boit number for radiation
    if condin == 0
        Fos1 = 0;
    else
        if (x(1)-dx1) <= 0
            dx1 = 0;
        end
        Fos1 = dt*k(1)/(rho(1)*Cp(1)*((x(2)-dx1/2)^2-x(1)^2)*log((x(1)/(x(1)-dx1)))); %Fourier number for conduction BC
    end
end
% form system arrays
B(1) = 0;
D(1) = 1 + Fo1 + Fo1*Bi1 + Fo1*BiRad1 + Fos1; %system array D
A(1) = -Fo1; %system array A
C(1) = (1 - Fo1 - Fo1*Bi1 - Fo1*BiRad1 - Fos1)*To(1) + Fo1*To(2) + 2*Fo1*Bi1*Tfin + 2*Fo1*BiRad1*Textin + 2*Fos1*Tsin; %system array C
% --- interior nodes
for i = 2:(n-1)
    % distance between nodes
    del1 = x(i) - x(i-1);
    del2 = x(i+1) - x(i);
    % simplification coefficients (for spatial discretization)
    C1 = 1 + (del1^3/del2^2 - del1)/(del2 + del1);
    C2 = 1 + (del1/del2)^3;
    C3 = (del1/del2)^3 - ((del1^3/del2^2) - del1)/(del2+del1);
    % calculated Fourier numbers
    Fo = 2*k(i)*dt/(rho(i)*Cp(i)*(del1^2 + del1^3/del2)); %Fourier number
    Fok = (dt/(rho(i)*Cp(i)*(del1+del2)))*((k(i+1)-k(i-1))/(del1+del2) + a*k(i)/x(i)); %Fourier number for conductivity variation and shape
    % adjust equations for change in materials
    %   when there is a change in materials the transition in materials
    %   properties, most notabely thermal conductivity, is abrupt. This
    %   discontinuty can cause accuracy and stability issues with the 
    %   derivative term dk/dt = (k(i+1)-k(i-1))/(del1+del2). Therefore a
    %   more robust approach is utilized when a material transition is
    %   detected. This method is document in "Integrated Turbine Tip
    %   Clearance and Gas Turbine Engine Simulation" by J. Chapman, J.
    %   Kratz, T.-H. Guo, and J. Litt. The method uses a transition Fourier
    %   number to address the discontinuity. The method from this reference
    %   has been generalized for non-uniform discretizations and geometries
    %   that could be either planar or cylindrical. When there is not a
    %   transition in materials the dk/dt term should be better
    %   approximated with the central difference scheme that is used and
    %   the standard formulation will be utilized. Material transition is
    %   detected by a sigificant (10%) increase or decrease in thermal 
    %   conductivity.
    if (k(i+1)/k(i)) > 1.1 || (k(i+1)/k(i)) < 0.9 %detect change in material
        Fo = k(i)*dt/(rho(i)*Cp(i)*dx(i)^2);
        Fok = (dt/(rho(i)*Cp(i)*(del1+del2)))*(a*k(i)/x(i));
        Fob = (k(i)*(dx(i)/2)+k(i+1)*(del2-dx(i)/2))*dt/(rho(i)*Cp(i)*del2*del1*del2);
        K1 = Fo;
        K2 = 2*0.5*(Fo+Fob); 
        K3 = Fob;
    elseif (k(i)/k(i-1)) > 1.1 || (k(i)/k(i-1)) < 0.9 %detect change in material
        Fo = k(i)*dt/(rho(i)*Cp(i)*dx(i)^2);
        Fok = (dt/(rho(i)*Cp(i)*(del1+del2)))*(a*k(i)/x(i));
        Foa = (k(i)*(dx(i)/2)+k(i-1)*(del1-dx(i)/2))*dt/(rho(i)*Cp(i)*del1*del1*del2);
        K1 = Foa;
        K2 = 2*0.5*(Fo+Foa); 
        K3 = Fo;
    else % no change in material detected - go with standard solution
        K1 = C1*Fo;
        K2 = C2*Fo;
        K3 = C3*Fo;
    end
    % form system arrays (B, D, A, and C)
    B(i) = 0.5*Fok - 0.5*K1;
    D(i) = 1 + 0.5*K2;
    A(i) = -0.5*Fok - 0.5*K3;
    C(i) = (-0.5*Fok+0.5*K1)*To(i-1) + (1-0.5*K2)*To(i) + (0.5*Fok+0.5*K3)*To(i+1);
end
% --- outer node (half size of interior node with point on surface)
Fon = 0; %Fourier number
Bin = 0; %Boit number
BiRadn = 0; %analogous Boit number for radiation
Fosn = 0; %Fourier number for conduction BC
dxn = x(n) - x(n-1); %node size
% planar
if a == 0
    Fon = dt*k(n)/(rho(n)*Cp(n)*dxn^2); %Fourier number
    Bin = hout*dxn/k(n); %Boit number
    BiRadn = uout*dxn/k(n); %analogous Boit number for radiation
    if condout == 0
        Fosn = 0;
    else
        Fosn = Fon; %Fourier number for conduction BC
    end
end
% cylindrical
if a == 1
    Fon = dt*k(n)/(rho(n)*Cp(n)*(x(n)^2-(x(n-1)+dxn/2)^2)*log(x(n)/x(n-1))); %Fourier number
    Bin = hout*x(n)*log(x(n)/x(n-1))/k(n); %Boit number
    BiRadn = uout*x(n)*log(x(n)/x(n-1))/k(n); %analogous Boit number for radiation
    if condout == 0
        Fosn = 0;
    else
        Fosn = dt*k(n)/(rho(n)*Cp(n)*(x(n)^2-(x(n-1)+dxn/2)^2)*log((x(n)+dxn)/x(n))); %Fourier number for conduction BC
    end
end
% form system arrays
D(n) = 1 + Fon + Fon*Bin + Fon*BiRadn + Fosn; %system array D
B(n) = -Fon; %system array B
A(n) = 0; %system array A
C(n) = (1 - Fon - Fon*Bin - Fon*BiRadn - Fosn)*To(n) + Fon*To(n-1) + 2*Fon*Bin*Tfout + 2*Fon*BiRadn*Textout + 2*Fosn*Tsout; %system array C

% solve for new temperatures using Thomas's Algorithm --------------------%
Dnew = zeros(1,n);
Cnew = zeros(1,n);
Dnew(1) = D(1);
Cnew(1) = C(1);
% build the rest of the new D-vector and C-vector using Guassian
% elimination
for i = 2:n
    Dnew(i) = D(i) - A(i-1)*B(i)/Dnew(i-1);
    Cnew(i) = C(i) - B(i)*Cnew(i-1)/Dnew(i-1);
end
% initialize the solution vector (i.e. the new temperature vector T)
T = zeros(1,n);
T(n) = Cnew(n)/Dnew(n);
for i = (n-1):-1:1
    T(i) = (Cnew(i) - A(i)*T(i+1))/Dnew(i);
end
